simulink model "q3_simulacao"  (Simulink 7.5)
settings: Solver=ode4  StartTime=0.0  StopTime=tempo_simulacao  FixedStep=0.8  RelTol=1e-3
values from neighbouring files (symbols this model uses):
  a = 1    [q3.m]
  a_m = 2    [q3.m]
  b = 1    [q3.m]
  b_m = 1    [q3.m]
  c = 1    [q3.m]
  c_m = 1    [q3.m]
  gamma = gammas( i )    [q3.m]
  periodo_ref = 200    [q3.m]
settings Model: Creator=diogo  LastModifiedBy=diogo

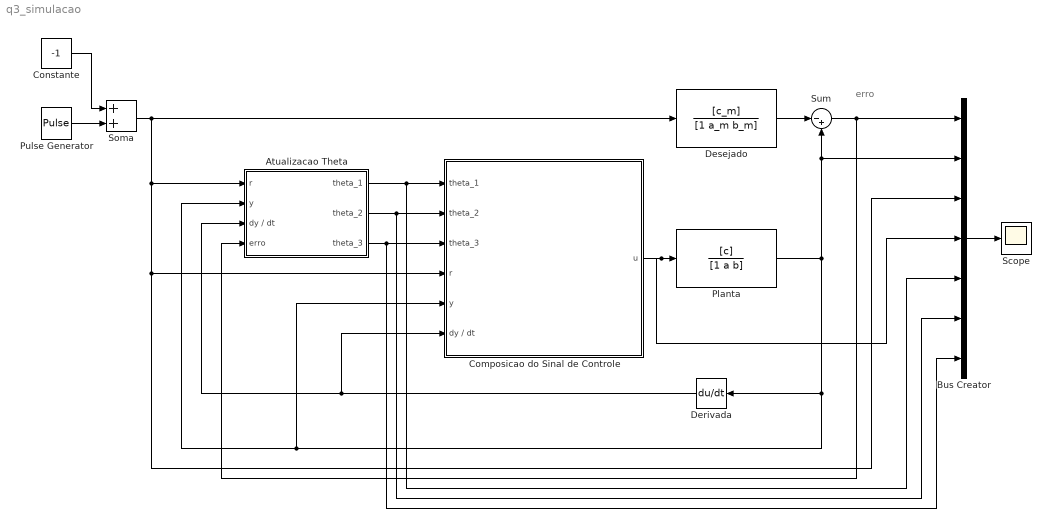
== system q3_simulacao ==
  note: erro
  Atualizacao Theta : Subsystem
  Bus Creator : BusCreator  Inputs=7
  Composicao do Sinal de Controle : Subsystem
  Constante : Constant  Value=-1  OutDataType=fixdt(1, 16)  OutScaling=2^0
  Derivada : Derivative
  Desejado : TransferFcn  Numerator=[c_m]  Denominator=[1 a_m b_m]
  Planta : TransferFcn  Numerator=[c]  Denominator=[1 a b]
  Pulse Generator : DiscretePulseGenerator  PulseType=Time based  Amplitude=2  Period=periodo_ref  PulseWidth=50  PhaseDelay=0  SampleTime=1
  Scope : Scope
      settings: YMax=1000  SaveName=saida  DataFormat=Array
  Soma : Sum  OutDataType=fixdt(1, 16)  OutScaling=2^-10
  Sum : Sum  Inputs=|-+  OutDataType=fixdt(1, 16)  OutScaling=2^0
  wires:
  Desejado/1 -> Sum/1
  Planta/1 -> Sum/2, Bus Creator/2, Atualizacao Theta/2(y), Composicao do Sinal de Controle/5(y), Derivada/1
  Sum/1 -> Bus Creator/1, Atualizacao Theta/4(erro)
  Composicao do Sinal de Controle/1(u) -> Planta/1, Bus Creator/4
  Atualizacao Theta/1(theta_1) -> Composicao do Sinal de Controle/1(theta_1), Bus Creator/5
  Atualizacao Theta/2(theta_2) -> Composicao do Sinal de Controle/2(theta_2), Bus Creator/6
  Atualizacao Theta/3(theta_3) -> Composicao do Sinal de Controle/3(theta_3), Bus Creator/7
  Bus Creator/1 -> Scope/1
  Derivada/1 -> Composicao do Sinal de Controle/6(dy / dt), Atualizacao Theta/3(dy / dt)
  Soma/1 -> Atualizacao Theta/1(r), Composicao do Sinal de Controle/4(r), Bus Creator/3, Desejado/1
  Constante/1 -> Soma/1
  Pulse Generator/1 -> Soma/2

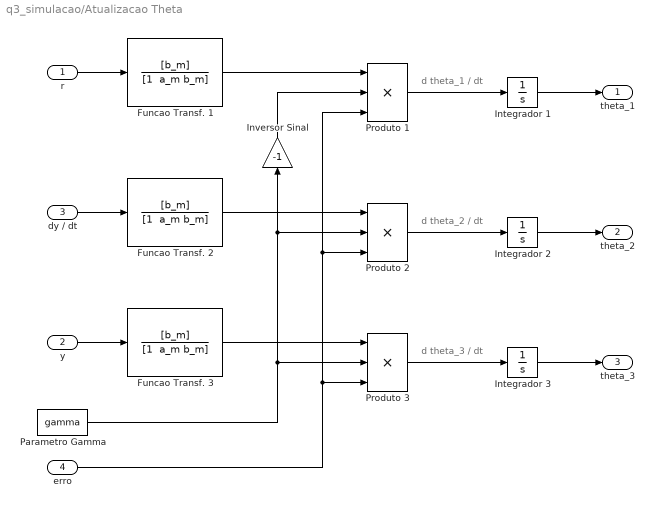
== system q3_simulacao/Atualizacao Theta ==
  note: d theta_1 / dt
  note: d theta_2 / dt
  note: d theta_3 / dt
  r : Inport  OutDataType=fixdt(1, 16)  OutScaling=2^0
  y : Inport  Port=2  OutDataType=fixdt(1, 16)  OutScaling=2^0
  dy / dt : Inport  Port=3  OutDataType=fixdt(1, 16)  OutScaling=2^0
  erro : Inport  Port=4  OutDataType=fixdt(1, 16)  OutScaling=2^0
  Funcao Transf. 1 : TransferFcn  Numerator=[b_m]  Denominator="[1  a_m b_m]"
  Funcao Transf. 2 : TransferFcn  Numerator=[b_m]  Denominator="[1  a_m b_m]"
  Funcao Transf. 3 : TransferFcn  Numerator=[b_m]  Denominator="[1  a_m b_m]"
  Integrador 1 : Integrator
  Integrador 2 : Integrator
  Integrador 3 : Integrator
  Inversor Sinal : Gain  Gain=-1  ParameterDataType=fixdt(1, 16)  ParameterScaling=2^0  OutDataType=fixdt(1, 16)  OutScaling=2^0
  Parametro Gamma : Constant  Value=gamma  OutDataType=fixdt(1, 16)  OutScaling=2^0
  Produto 1 : Product  Inputs=3  OutDataType=fixdt(1, 16)  OutScaling=2^0  RndMeth=Zero
  Produto 2 : Product  Inputs=3  OutDataType=fixdt(1, 16)  OutScaling=2^0  RndMeth=Zero
  Produto 3 : Product  Inputs=3  OutDataType=fixdt(1, 16)  OutScaling=2^0  RndMeth=Zero
  theta_1 : Outport  OutDataType=fixdt(1, 16)  OutScaling=2^0
  theta_2 : Outport  Port=2  OutDataType=fixdt(1, 16)  OutScaling=2^0
  theta_3 : Outport  Port=3  OutDataType=fixdt(1, 16)  OutScaling=2^0
  wires:
  r/1 -> Funcao Transf. 1/1
  y/1 -> Funcao Transf. 3/1
  Produto 1/1 -> Integrador 1/1
  Produto 2/1 -> Integrador 2/1
  Integrador 1/1 -> theta_1/1
  Integrador 2/1 -> theta_2/1
  Integrador 3/1 -> theta_3/1
  Produto 3/1 -> Integrador 3/1
  Inversor Sinal/1 -> Produto 1/2
  Parametro Gamma/1 -> Inversor Sinal/1, Produto 2/2, Produto 3/2
  Funcao Transf. 1/1 -> Produto 1/1
  Funcao Transf. 2/1 -> Produto 2/1
  Funcao Transf. 3/1 -> Produto 3/1
  dy / dt/1 -> Funcao Transf. 2/1
  erro/1 -> Produto 1/3, Produto 2/3, Produto 3/3

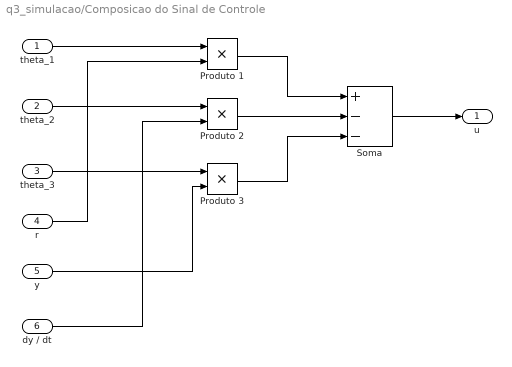
== system q3_simulacao/Composicao do Sinal de Controle ==
  theta_1 : Inport  OutDataType=fixdt(1, 16)  OutScaling=2^0
  theta_2 : Inport  Port=2  OutDataType=fixdt(1, 16)  OutScaling=2^0
  theta_3 : Inport  Port=3  OutDataType=fixdt(1, 16)  OutScaling=2^0
  r : Inport  Port=4  OutDataType=fixdt(1, 16)  OutScaling=2^0
  y : Inport  Port=5  OutDataType=fixdt(1, 16)  OutScaling=2^0
  dy / dt : Inport  Port=6  OutDataType=fixdt(1, 16)  OutScaling=2^0
  Produto 1 : Product  OutDataType=fixdt(1, 16)  OutScaling=2^0  RndMeth=Zero
  Produto 2 : Product  OutDataType=fixdt(1, 16)  OutScaling=2^0  RndMeth=Zero
  Produto 3 : Product  OutDataType=fixdt(1, 16)  OutScaling=2^0  RndMeth=Zero
  Soma : Sum  Inputs=+--  OutDataType=fixdt(1, 16)  OutScaling=2^-10
  u : Outport  OutDataType=fixdt(1, 16)  OutScaling=2^0
  wires:
  Soma/1 -> u/1
  theta_1/1 -> Produto 1/1
  r/1 -> Produto 1/2
  theta_2/1 -> Produto 2/1
  dy / dt/1 -> Produto 2/2
  theta_3/1 -> Produto 3/1
  y/1 -> Produto 3/2
  Produto 2/1 -> Soma/2
  Produto 1/1 -> Soma/1
  Produto 3/1 -> Soma/3
